simulink model "torch_zdof_sim"  (R2025b)
settings: Solver=VariableStepAuto  StartTime=0.0  StopTime=267.8481  RelTol=1e-3
values from neighbouring files (symbols this model uses):
  framePeriod_s = 1/frameRate_hz    (= 0.005)    [setup.m]
  frameRate_hz = 200    [setup.m]
undefined symbols (not defined in the file or in its folder): Aircraft
libraries: simulink x11, slpidlib x3, uavutilslib x1
settings Model: Creator=amark  LastModifiedBy=zpowe
settings RTWCC: GenCodeOnly=on  Toolchain=MinGW64 | gmake (64-bit Windows)

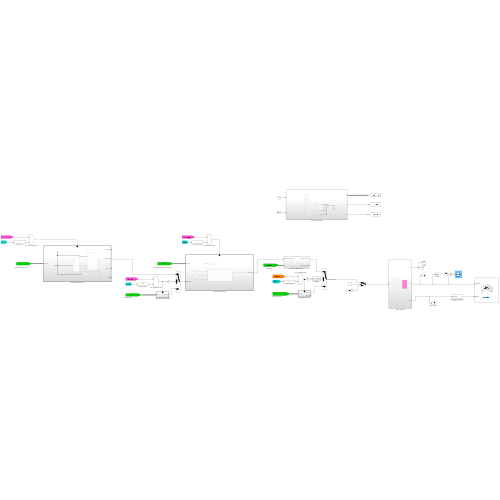
[thumbnail: Simulink's stored preview of the top-level diagram]
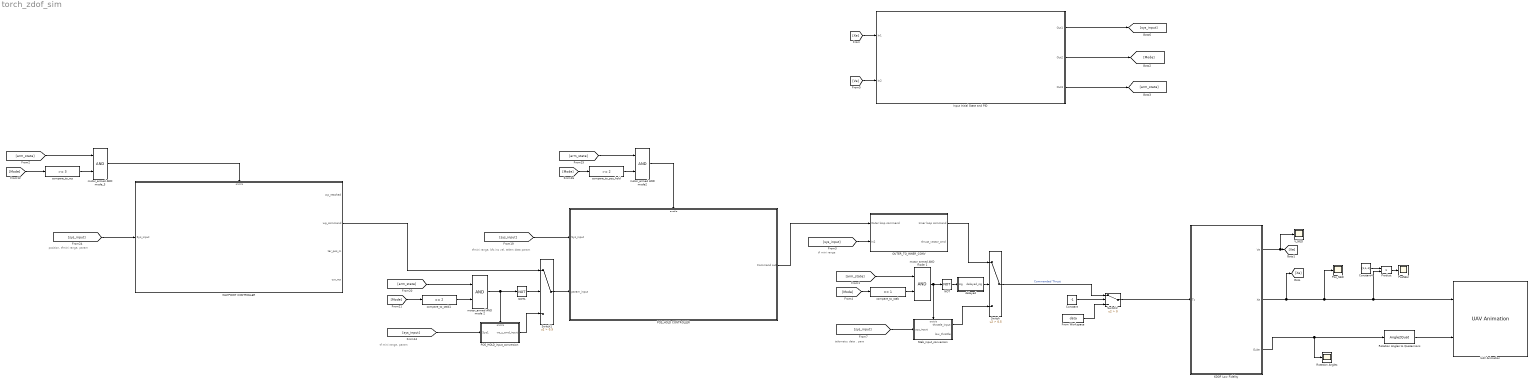
== system torch_zdof_sim ==
  note: position, tfmini range, param
  note: tf mini range, param
  note: tfmini range, bfs ins vel, telem data param
  note: telemetry data . para
  note: tf mini range
  6DOF Low Fidelity : Subsystem
  Constant : Constant  Value=-1
  Constant4 : Constant  Value=[1,1,-1]
  From Workspace : FromWorkspace  VariableName=data  SampleTime=0.005
  Input Initial State and PID : Subsystem
  NOT : Logic  Operator=NOT  IconShape=distinctive  AllPortsSameDT=off  OutDataTypeStr=boolean
  NOT1 : Logic  Operator=NOT  IconShape=distinctive  AllPortsSameDT=off  OutDataTypeStr=boolean
  OUTER_TO_INNER_CONV : Subsystem
  POS_HOLD CONTROLLER : Subsystem
  POS_HOLD_input_conversion : Subsystem
  PosNEU : Scope
      settings: ActiveDisplayYMinimum=-0.21626329278447132  ActiveDisplayYMaximum=2.0187949768508888
  Pos_NED : Scope
      settings: ActiveDisplayYMinimum=-8.6714235476794528  ActiveDisplayYMaximum=15.654477836769015  DataLoggingVariableName=ScopeData7
  Product : Product
  Rotation Angles : Scope
      settings: ActiveDisplayYMinimum=-3.621315177012066  ActiveDisplayYMaximum=3.4944012677530658  DataLoggingVariableName=ScopeData3
  Rotation Angles to Quaternions : Angle2Quat  rotationOrder=XYZ
      settings: AttributesFormatString=Rotation Order: %<rotationOrder>
  Stab_input_conversion : Subsystem
  Switch : Switch  Criteria=u2 > Threshold  Threshold=0.5  SaturateOnIntegerOverflow=off  InputSameDT=off
  Switch1 : Switch  Criteria=u2 > Threshold  Threshold=0.5  SaturateOnIntegerOverflow=off  InputSameDT=off
  Switch2 : Switch  Criteria=u2 > Threshold  SaturateOnIntegerOverflow=off  InputSameDT=off
  UAV Animation : uavutilslib/UAV Animation  NumUAV=1  DynamicUAVConfig=off  UAVType=Multirotor  UAVSize=1  UAVColor=[1 0 0]  UAVTrajectoryAlpha=1  InertialZDirection=Down  RotationFormat=Quaternion  DrawMarkers=off  SampleTime=0.5
  V_NED : Scope
      settings: ActiveDisplayYMinimum=-0.923125150146191  ActiveDisplayYMaximum=0.89093380676990863  DataLoggingVariableName=ScopeData2
  WAYPOINT CONTROLLER : Subsystem
  compare_to_pos_hold : simulink/Logic and Bit Operations/Compare To Constant  relop=>=  const=2  OutDataTypeStr=boolean
  compare_to_stab : simulink/Logic and Bit Operations/Compare To Constant  relop===  const=1  OutDataTypeStr=boolean
  compare_to_stab1 : simulink/Logic and Bit Operations/Compare To Constant  relop===  const=2  OutDataTypeStr=boolean
  compare_to_wp : simulink/Logic and Bit Operations/Compare To Constant  relop=>=  const=3  OutDataTypeStr=boolean
  delayed : Subsystem
  motor_armed AND mode 1 : Logic  IconShape=distinctive  AllPortsSameDT=off  OutDataTypeStr=boolean
  motor_armed AND mode 2 : Logic  IconShape=distinctive  AllPortsSameDT=off  OutDataTypeStr=boolean
  motor_armed AND mode2 : Logic  IconShape=distinctive  AllPortsSameDT=off  OutDataTypeStr=boolean
  motor_armed AND mode_3 : Logic  IconShape=distinctive  AllPortsSameDT=off  OutDataTypeStr=boolean
  wires:
  6DOF Low Fidelity/2(Xe) -> [Xe], UAV Animation/1, Product/2, Pos_NED/1
  6DOF Low Fidelity/1(Ve) -> V_NED/1, [Ve]
  6DOF Low Fidelity/3(Euler) -> Rotation Angles to Quaternions/1, Rotation Angles/1
  Constant4/1 -> Product/1
  Product/1 -> PosNEU/1
  Rotation Angles to Quaternions/1 -> UAV Animation/2
  [sys_input] -> POS_HOLD CONTROLLER/1(Sys_input)
  compare_to_pos_hold/1 -> motor_armed AND mode2/2
  compare_to_wp/1 -> motor_armed AND mode_3/2
  compare_to_stab1/1 -> motor_armed AND mode 2/2
  motor_armed AND mode 2/1 -> NOT1/1, POS_HOLD_input_conversion/Enable
  [arm_state] -> motor_armed AND mode 1/1
  POS_HOLD CONTROLLER/1(Command out) -> OUTER_TO_INNER_CONV/1(Outer loop command)
  compare_to_stab/1 -> motor_armed AND mode 1/2
  [Mode] -> compare_to_wp/1
  [arm_state] -> motor_armed AND mode2/1
  Switch1/1 -> POS_HOLD CONTROLLER/2(param_input)
  Stab_input_conversion/1(throttle_input) -> Switch/3
  [Mode] -> compare_to_stab1/1
  NOT1/1 -> Switch1/2
  [sys_input] -> POS_HOLD_input_conversion/1(Sys1)
  WAYPOINT CONTROLLER/2(wp_command) -> Switch1/1
  [sys_input] -> Stab_input_conversion/1(sys_input)
  delayed/1(delayed_sig) -> Switch/2
  motor_armed AND mode_3/1 -> WAYPOINT CONTROLLER/Enable
  POS_HOLD_input_conversion/1(ve_z_cmd_input) -> Switch1/3
  [arm_state] -> motor_armed AND mode 2/1
  [sys_input] -> OUTER_TO_INNER_CONV/2(In2)
  [sys_input] -> WAYPOINT CONTROLLER/1(Sys_input)
  [Mode] -> compare_to_pos_hold/1
  NOT/1 -> delayed/1(sig)
  [arm_state] -> motor_armed AND mode_3/1
  OUTER_TO_INNER_CONV/1(Inner loop command) -> Switch/1
  motor_armed AND mode 1/1 -> NOT/1, Stab_input_conversion/Enable
  [Mode] -> compare_to_stab/1
  motor_armed AND mode2/1 -> POS_HOLD CONTROLLER/Enable
  Input Initial State and PID/1(Out1) -> [sys_input]
  Input Initial State and PID/2(Out2) -> [Mode]
  Input Initial State and PID/3(Out3) -> [arm_state]
  [Ve] -> Input Initial State and PID/2(In2)
  [Xe] -> Input Initial State and PID/1(In1)
  From Workspace/1 -> Switch2/3
  Switch2/1 -> 6DOF Low Fidelity/1(Tz)
  Constant/1 -> Switch2/2
  Switch/1 -> Switch2/1  "Commanded Thrust"

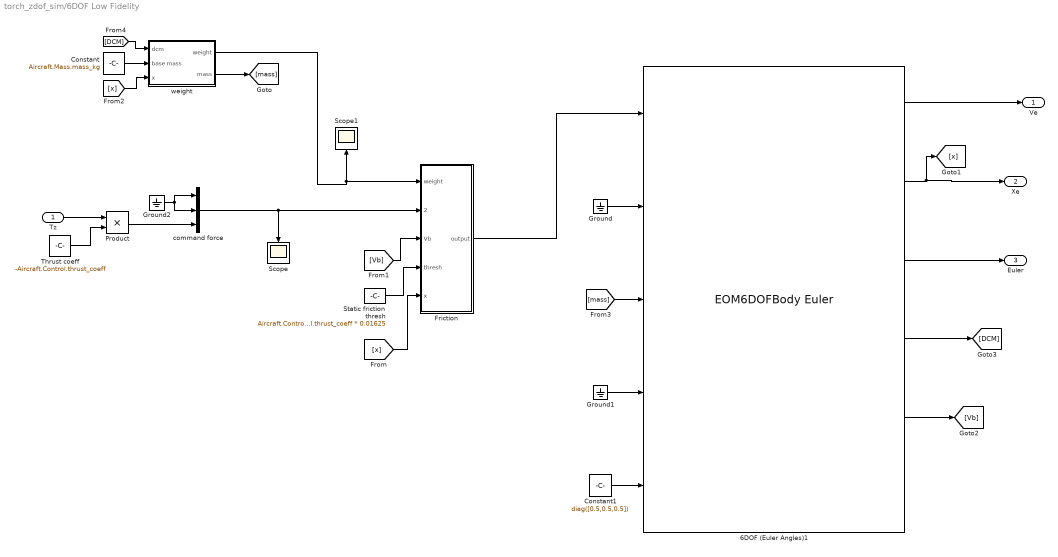
== system torch_zdof_sim/6DOF Low Fidelity ==
  Tz : Inport
  " command force" : Mux  Inputs=3
  6DOF (Euler Angles)1 : EOM6DOFBodyEuler  mtype=Custom Variable  mass_0=Aircraft.Mass.mass_kg  inertia=diag([3.2e-4,100,100])  mass_flag=on
  Constant : Constant  Value=Aircraft.Mass.mass_kg
  Constant1 : Constant  Value=diag([0.5,0.5,0.5])
  Friction : MATLAB Function  TreatAsAtomicUnit=on
  Ground : Ground
  Ground1 : Ground
  Ground2 : Ground
  Product : Product
  Scope : Scope
      settings: ActiveDisplayYMinimum=-1  ActiveDisplayYMaximum=1  DataLoggingVariableName=ScopeData5
  Scope1 : Scope
      settings: ActiveDisplayYMinimum=-12.429607540477818  ActiveDisplayYMaximum=125.41660771198916  DataLoggingVariableName=ScopeData6
  Static friction thresh : Constant  Value=Aircraft.Control.thrust_coeff * 0.01625
  Thrust coeff : Constant  Value=-Aircraft.Control.thrust_coeff
  weight : Subsystem
  Ve : Outport
  Xe : Outport  Port=2
  Euler : Outport  Port=3
  wires:
  6DOF (Euler Angles)1/2 -> [x], Xe/1
  6DOF (Euler Angles)1/3 -> Euler/1
  6DOF (Euler Angles)1/1 -> Ve/1
  6DOF (Euler Angles)1/5 -> [Vb]
  6DOF (Euler Angles)1/4 -> [DCM]
  weight/1(weight) -> Scope1/1, Friction/1(weight)
  " command force"/1 -> Scope/1, Friction/2(F_command)
  [DCM] -> weight/1(dcm)
  [Vb] -> Friction/3(Vb)
  Ground2/1 -> " command force"/2, " command force"/1
  Friction/1(output) -> 6DOF (Euler Angles)1/1
  Tz/1 -> Product/1
  Static friction thresh/1 -> Friction/4(thresh)
  Constant/1 -> weight/2(base mass)
  [x] -> weight/3(x)
  Product/1 -> " command force"/3
  Thrust coeff/1 -> Product/2
  Ground/1 -> 6DOF (Euler Angles)1/2
  [x] -> Friction/5(x)
  Ground1/1 -> 6DOF (Euler Angles)1/4
  weight/2(mass) -> [mass]
  [mass] -> 6DOF (Euler Angles)1/3
  Constant1/1 -> 6DOF (Euler Angles)1/5

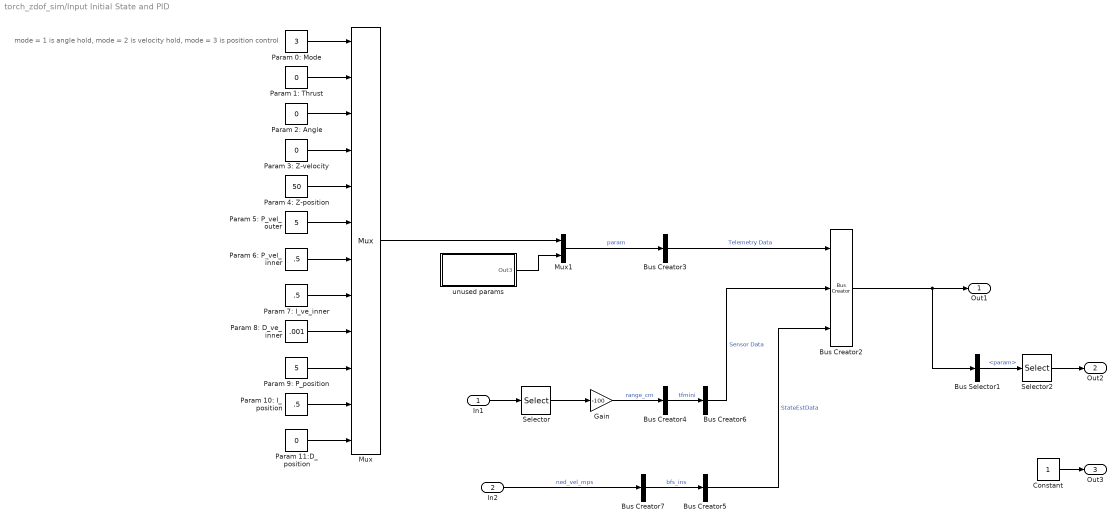
== system torch_zdof_sim/Input Initial State and PID ==
  note: mode = 1 is angle hold, mode = 2 is velocity hold, mode = 3 is position control
  In1 : Inport
  In2 : Inport  Port=2
  Bus Creator2 : BusCreator  Inputs=3
  Bus Creator{3..7} (5 alike) : BusCreator  Inputs=1
  Bus Selector1 : BusSelector  OutputSignals=Telemetry Data.param
  Constant : Constant
  Gain : Gain  Gain=-100
  Mux : Mux  Inputs=12
  Mux1 : Mux  Inputs=2
  Param 0: Mode : Constant  Value=3
  Param 10: I_position : Constant  Value=.5
  Param 11:D_position : Constant  Value=0
  Param 1: Thrust : Constant  Value=0
  Param 2: Angle : Constant  Value=0
  Param 3: Z-velocity : Constant  Value=0
  Param 4: Z-position : Constant  Value=50
  Param 5: P_vel_outer : Constant  Value=5
  Param 6: P_vel_inner : Constant  Value=.5
  Param 7: I_ve_inner : Constant  Value=.5
  Param 8: D_ve_inner : Constant  Value=.001
  Param 9: P_position : Constant  Value=5
  Selector : Selector  InputPortWidth=3  IndexOptions=Index vector (dialog)  Indices=[3]  OutputSizes=1
  Selector2 : Selector  IndexMode=Zero-based  InputPortWidth=24  IndexOptions=Index vector (dialog)  Indices=0  OutputSizes=1
  unused params : Subsystem
  Out1 : Outport
  Out2 : Outport  Port=2
  Out3 : Outport  Port=3
  wires:
  Param 3: Z-velocity/1 -> Mux/4
  Bus Creator5/1 -> Bus Creator2/3  "StateEstData"
  Param 2: Angle/1 -> Mux/3
  Param 4: Z-position/1 -> Mux/5
  Selector/1 -> Gain/1
  Param 11:D_position/1 -> Mux/12
  Param 10: I_position/1 -> Mux/11
  Param 9: P_position/1 -> Mux/10
  Bus Creator6/1 -> Bus Creator2/2  "Sensor Data"
  Param 7: I_ve_inner/1 -> Mux/8
  Param 1: Thrust/1 -> Mux/2
  Param 5: P_vel_outer/1 -> Mux/6
  Bus Creator4/1 -> Bus Creator6/1  "tfmini"
  Bus Creator3/1 -> Bus Creator2/1  "Telemetry Data"
  Param 8: D_ve_inner/1 -> Mux/9
  Param 0: Mode/1 -> Mux/1
  Gain/1 -> Bus Creator4/1  "range_cm"
  Param 6: P_vel_inner/1 -> Mux/7
  In1/1 -> Selector/1
  In2/1 -> Bus Creator7/1  "ned_vel_mps"
  Mux/1 -> Mux1/1
  Bus Creator7/1 -> Bus Creator5/1  "bfs_ins"
  Bus Selector1/1 -> Selector2/1  "<param>"
  Bus Creator2/1 -> Bus Selector1/1, Out1/1
  Selector2/1 -> Out2/1
  Constant/1 -> Out3/1
  Mux1/1 -> Bus Creator3/1  "param"
  unused params/1(Out3) -> Mux1/2

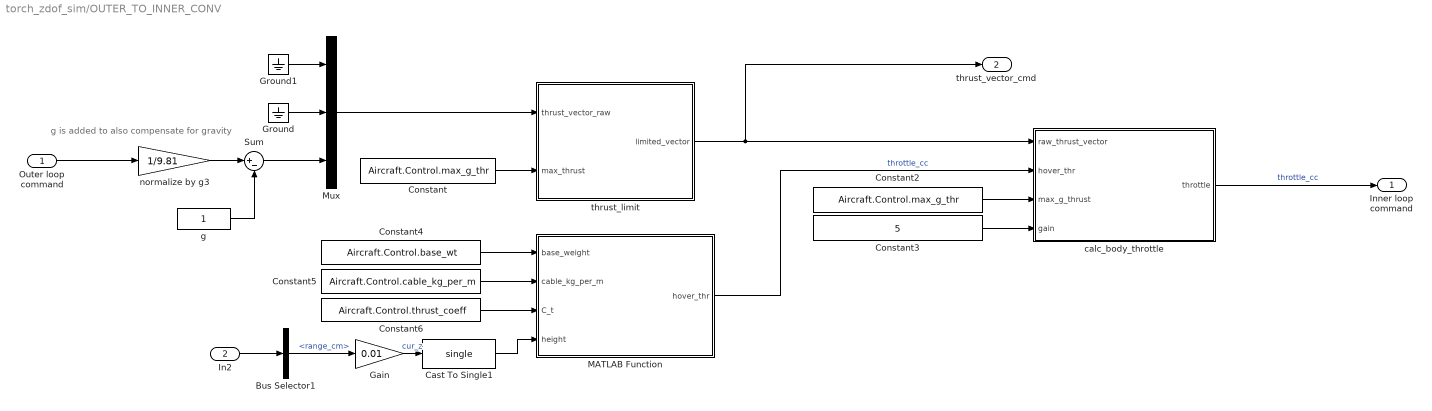
== system torch_zdof_sim/OUTER_TO_INNER_CONV ==
  note: g is added to also compensate for gravity
  Outer loop command : Inport
  In2 : Inport  Port=2
  Bus Selector1 : BusSelector  OutputSignals=Sensor Data.tfmini.range_cm
  Cast To Single1 : DataTypeConversion  OutDataTypeStr=single  SaturateOnIntegerOverflow=off  RndMeth=Floor
  Constant : Constant  Value=Aircraft.Control.max_g_thr  OutDataTypeStr=single
  Constant2 : Constant  Value=Aircraft.Control.max_g_thr  OutDataTypeStr=single
  Constant3 : Constant  Value=5  OutDataTypeStr=single
  Constant4 : Constant  Value=Aircraft.Control.base_wt  OutDataTypeStr=double
  Constant5 : Constant  Value=Aircraft.Control.cable_kg_per_m  OutDataTypeStr=double
  Constant6 : Constant  Value=Aircraft.Control.thrust_coeff  OutDataTypeStr=double
  Gain : Gain  Gain=0.01
  Ground : Ground
  Ground1 : Ground
  MATLAB Function : MATLAB Function  TreatAsAtomicUnit=on
  Mux : Mux  Inputs=3
  Sum : Sum  Inputs=|+-
  calc_body_throttle : MATLAB Function  TreatAsAtomicUnit=on
  g : Constant  OutDataTypeStr=single
  normalize by g3 : Gain  Gain=1/9.81
  thrust_limit : MATLAB Function  TreatAsAtomicUnit=on
  Inner loop command : Outport
  thrust_vector_cmd : Outport  Port=2
  wires:
  Constant/1 -> thrust_limit/2(max_thrust)
  Mux/1 -> thrust_limit/1(thrust_vector_raw)
  Outer loop command/1 -> normalize by g3/1
  g/1 -> Sum/2
  normalize by g3/1 -> Sum/1
  Ground1/1 -> Mux/1
  Ground/1 -> Mux/2
  Sum/1 -> Mux/3
  calc_body_throttle/1(throttle) -> Inner loop command/1  "throttle_cc"
  thrust_limit/1(limited_vector) -> calc_body_throttle/1(raw_thrust_vector), thrust_vector_cmd/1
  Constant2/1 -> calc_body_throttle/3(max_g_thrust)
  Constant3/1 -> calc_body_throttle/4(gain)
  Constant5/1 -> MATLAB Function/2(cable_kg_per_m)
  In2/1 -> Bus Selector1/1
  Bus Selector1/1 -> Gain/1  "<range_cm>"
  Constant6/1 -> MATLAB Function/3(C_t)
  MATLAB Function/1(hover_thr) -> calc_body_throttle/2(hover_thr)  "throttle_cc"
  Cast To Single1/1 -> MATLAB Function/4(height)
  Gain/1 -> Cast To Single1/1  "cur_z"
  Constant4/1 -> MATLAB Function/1(base_weight)

== system torch_zdof_sim/POS_HOLD CONTROLLER ==
  Sys_input : Inport
  param_input : Inport  Port=2
  Enable : EnablePort  StatesWhenEnabling=reset  PropagateVarSize=During execution  ShowOutputPort=on
  Vertical speed controller : Subsystem
  Command out : Outport
  wires:
  Enable/1 -> [pos_hold_init]
  Vertical speed controller/1(acc_z_cmd) -> Command out/1  "acc_z_cmd"
  Sys_input/1 -> Vertical speed controller/3(sys_data)
  [pos_hold_init] -> Vertical speed controller/2(pos_hold_init)
  param_input/1 -> Vertical speed controller/1(ve_z_cmd_mps)

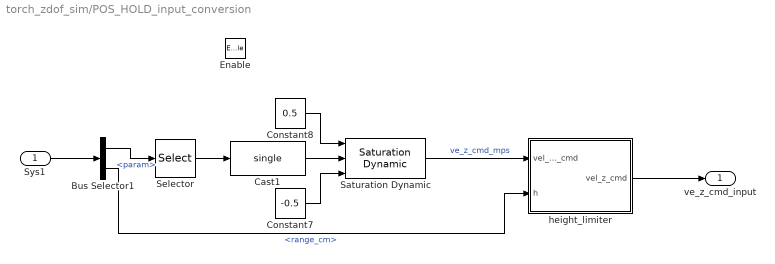
== system torch_zdof_sim/POS_HOLD_input_conversion ==
  Sys1 : Inport
  Enable : EnablePort
  Bus Selector1 : BusSelector  OutputSignals=Telemetry Data.param,Sensor Data.tfmini.range_cm
  Cast1 : DataTypeConversion  OutDataTypeStr=single  SaturateOnIntegerOverflow=off  RndMeth=Floor
  Constant7 : Constant  Value=-0.5
  Constant8 : Constant  Value=0.5
  Saturation Dynamic : simulink/Discontinuities/Saturation Dynamic  OutMin=[]  OutMax=[]  OutDataTypeStr=double  OutDataType=fixdt(1, 16)  OutScaling=2^-10  DoSatur=off
  Selector : Selector  IndexMode=Zero-based  InputPortWidth=24  IndexOptions=Index vector (dialog)  Indices=3  OutputSizes=1
  height_limiter : MATLAB Function  TreatAsAtomicUnit=on
  ve_z_cmd_input : Outport
  wires:
  Sys1/1 -> Bus Selector1/1
  Constant8/1 -> Saturation Dynamic/1
  Constant7/1 -> Saturation Dynamic/3
  Bus Selector1/1 -> Selector/1  "<param>"
  Cast1/1 -> Saturation Dynamic/2
  Selector/1 -> Cast1/1
  Saturation Dynamic/1 -> height_limiter/1(vel_param_cmd)  "ve_z_cmd_mps"
  Bus Selector1/2 -> height_limiter/2(h)  "<range_cm>"
  height_limiter/1(vel_z_cmd) -> ve_z_cmd_input/1

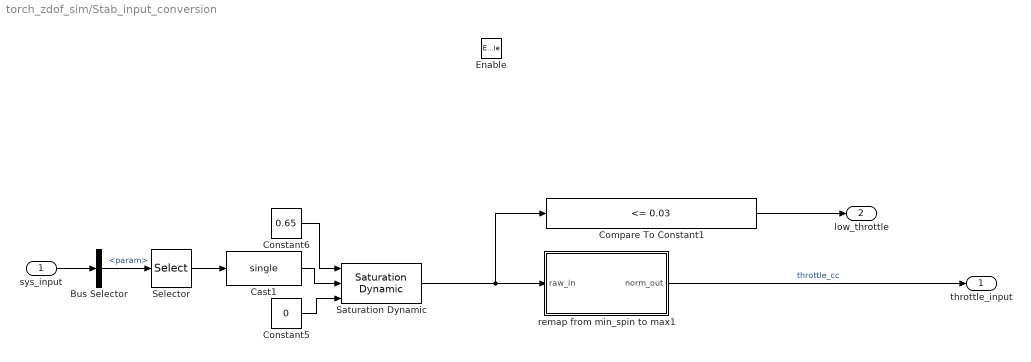
== system torch_zdof_sim/Stab_input_conversion ==
  sys_input : Inport
  Enable : EnablePort
  Bus Selector : BusSelector  OutputSignals=Telemetry Data.param
  Cast1 : DataTypeConversion  OutDataTypeStr=single  SaturateOnIntegerOverflow=off  RndMeth=Floor
  Compare To Constant1 : simulink/Logic and Bit Operations/Compare To Constant  relop=<=  const=0.03  OutDataTypeStr=boolean
  Constant5 : Constant  Value=0
  Constant6 : Constant  Value=0.65
  Saturation Dynamic : simulink/Discontinuities/Saturation Dynamic  OutMin=[]  OutMax=[]  OutDataTypeStr=double  OutDataType=fixdt(1, 16)  OutScaling=2^-10  DoSatur=off
  Selector : Selector  IndexMode=Zero-based  InputPortWidth=24  IndexOptions=Index vector (dialog)  Indices=1  OutputSizes=1
  remap from min_spin to max1 : Subsystem
  throttle_input : Outport
  low_throttle : Outport  Port=2
  wires:
  Compare To Constant1/1 -> low_throttle/1
  Constant6/1 -> Saturation Dynamic/1
  sys_input/1 -> Bus Selector/1
  Cast1/1 -> Saturation Dynamic/2
  Selector/1 -> Cast1/1
  Constant5/1 -> Saturation Dynamic/3
  Bus Selector/1 -> Selector/1  "<param>"
  Saturation Dynamic/1 -> Compare To Constant1/1, remap from min_spin to max1/1(raw_in)
  remap from min_spin to max1/1(norm_out) -> throttle_input/1  "throttle_cc"

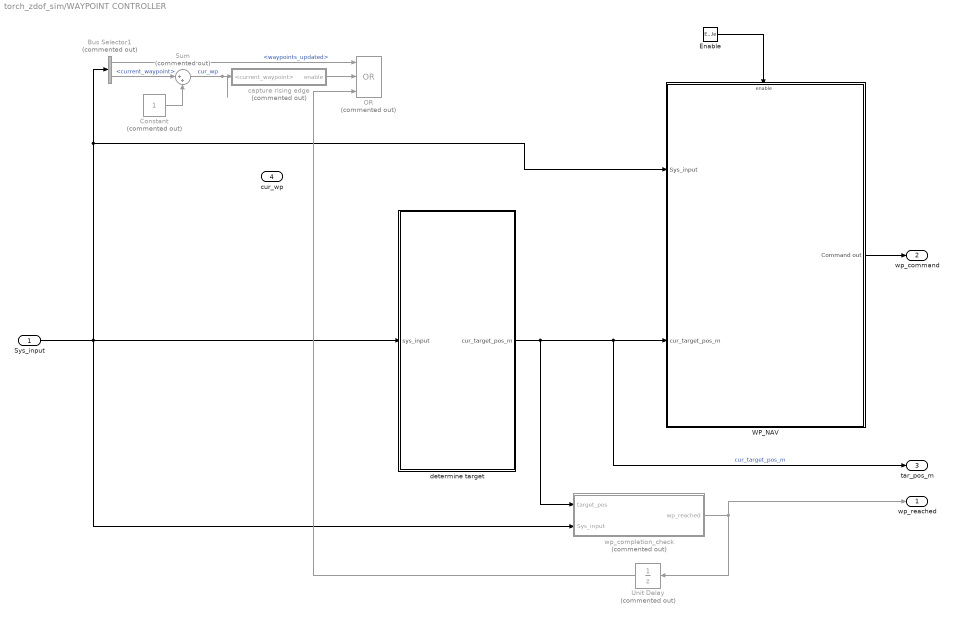
== system torch_zdof_sim/WAYPOINT CONTROLLER ==
  Sys_input : Inport
  Enable : EnablePort  StatesWhenEnabling=reset  ShowOutputPort=on
  Bus Selector1 : BusSelector  Commented=on  OutputSignals=Telemetry Data.waypoints_updated,Telemetry Data.current_waypoint
  Constant : Constant  Commented=on  OutDataTypeStr=int16
  OR : Logic  Commented=on  Operator=OR  Inputs=3  IconShape=distinctive  AllPortsSameDT=off  OutDataTypeStr=boolean
  Sum : Sum  Commented=on  Inputs=|++
  Unit Delay : UnitDelay  Commented=on  SampleTime=-1  HasFrameUpgradeWarning=on
  WP_NAV : Subsystem
  capture rising edge : Subsystem  Commented=on
  determine target : Subsystem
  wp_completion_check : Subsystem  Commented=on
  wp_reached : Outport
  wp_command : Outport  Port=2
  tar_pos_m : Outport  Port=3
  cur_wp : Outport  Port=4
  wires:
  Sys_input/1 -> Bus Selector1/1, WP_NAV/1(Sys_input), wp_completion_check/2(Sys_input), determine target/1(sys_input)
  Enable/1 -> WP_NAV/Enable
  WP_NAV/1(Command out) -> wp_command/1
  determine target/1(cur_target_pos_m) -> tar_pos_m/1, WP_NAV/2(cur_target_pos_m), wp_completion_check/1(target_pos)  "cur_target_pos_m"
  Bus Selector1/1 -> OR/1  "<waypoints_updated>"
  capture rising edge/1(enable) -> OR/2
  Unit Delay/1 -> OR/3
  wp_completion_check/1(wp_reached) -> wp_reached/1, Unit Delay/1
  Constant/1 -> Sum/2
  Bus Selector1/2 -> Sum/1  "<current_waypoint>"
  Sum/1 -> capture rising edge/1(<current_waypoint>)  "cur_wp"

== system torch_zdof_sim/delayed ==
  sig : Inport
  Constant : Constant  Value=framePeriod_s  OutDataTypeStr=double
  Constant1 : Constant  Value=0.5  OutDataTypeStr=single
  Delay : Delay  DelayLengthSource=Input port
      settings: InputPortMap=u0,p1
  Divide : Product  Inputs=*/
  delayed_sig : Outport
  wires:
  Delay/1 -> delayed_sig/1
  sig/1 -> Delay/1
  Divide/1 -> Delay/2
  Constant/1 -> Divide/2
  Constant1/1 -> Divide/1

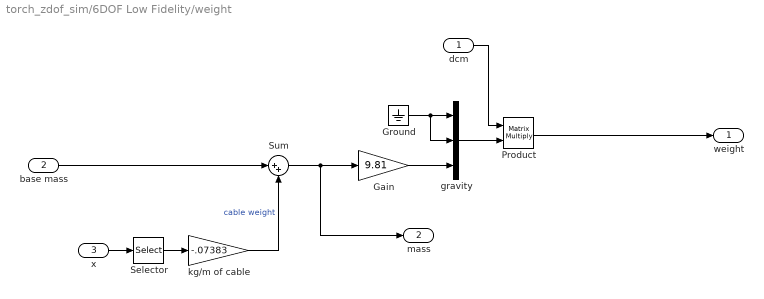
== system torch_zdof_sim/6DOF Low Fidelity/weight ==
  dcm : Inport
  base mass : Inport  Port=2
  x : Inport  Port=3
  Gain : Gain  Gain=9.81
  Ground : Ground
  Product : Product  Multiplication=Matrix(*)
  Selector : Selector  InputPortWidth=3  IndexOptions=Index vector (dialog)  Indices=[3]  OutputSizes=1
  Sum : Sum  Inputs=|++
  gravity : Mux  Inputs=3
  kg/m of cable : Gain  Gain=-.07383
  weight : Outport
  mass : Outport  Port=2
  wires:
  Ground/1 -> gravity/2, gravity/1
  gravity/1 -> Product/2
  base mass/1 -> Sum/1
  dcm/1 -> Product/1
  Gain/1 -> gravity/3
  Product/1 -> weight/1
  Sum/1 -> mass/1, Gain/1
  x/1 -> Selector/1
  Selector/1 -> kg/m of cable/1
  kg/m of cable/1 -> Sum/2  "cable weight"

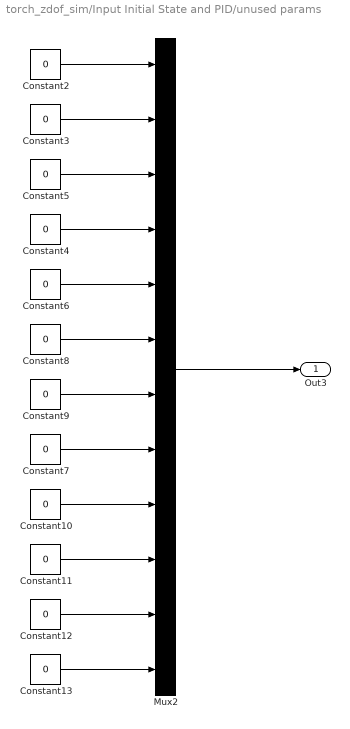
== system torch_zdof_sim/Input Initial State and PID/unused params ==
  Constant{2..13} (12 alike) : Constant  Value=0
  Mux2 : Mux  Inputs=12
  Out3 : Outport
  wires:
  Mux2/1 -> Out3/1
  Constant13/1 -> Mux2/12
  Constant12/1 -> Mux2/11
  Constant11/1 -> Mux2/10
  Constant10/1 -> Mux2/9
  Constant9/1 -> Mux2/7
  Constant8/1 -> Mux2/6
  Constant7/1 -> Mux2/8
  Constant6/1 -> Mux2/5
  Constant5/1 -> Mux2/3
  Constant4/1 -> Mux2/4
  Constant3/1 -> Mux2/2
  Constant2/1 -> Mux2/1

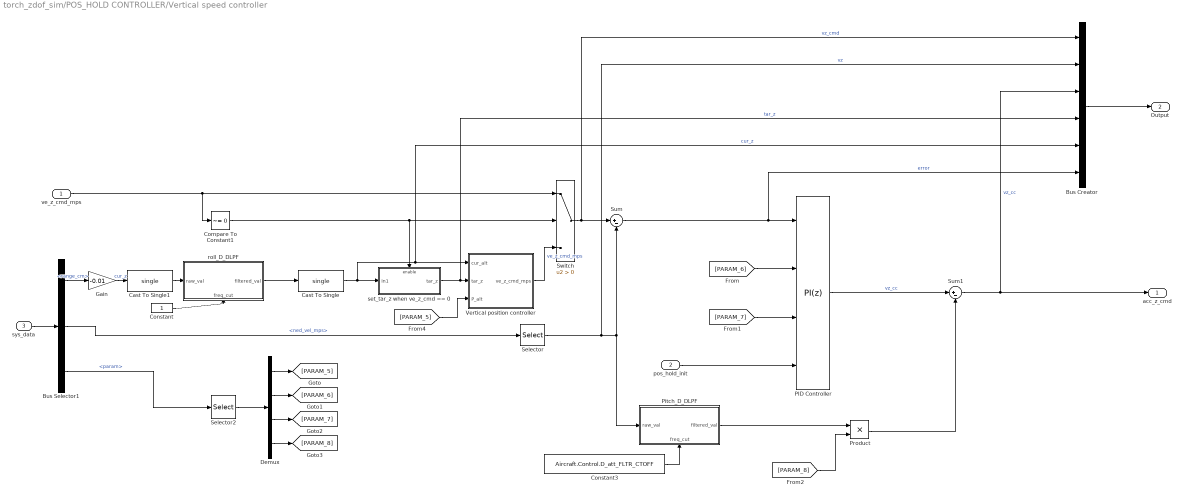
== system torch_zdof_sim/POS_HOLD CONTROLLER/Vertical speed controller ==
  ve_z_cmd_mps : Inport
  pos_hold_init : Inport  Port=2
  sys_data : Inport  Port=3
  Bus Creator : BusCreator  Inputs=6
  Bus Selector1 : BusSelector  OutputSignals=Sensor Data.tfmini.range_cm,StateEstData.bfs_ins.ned_vel_mps,Telemetry Data.param
  Cast To Single : DataTypeConversion  OutDataTypeStr=single  SaturateOnIntegerOverflow=off  RndMeth=Floor
  Cast To Single1 : DataTypeConversion  OutDataTypeStr=single  SaturateOnIntegerOverflow=off  RndMeth=Floor
  Compare To Constant1 : simulink/Logic and Bit Operations/Compare To Constant  relop=~=  const=0  OutDataTypeStr=boolean
  Constant : Constant  OutDataTypeStr=single
  Constant3 : Constant  Value=Aircraft.Control.D_att_FLTR_CTOFF  OutDataTypeStr=single
  Demux : Demux
  Gain : Gain  Gain=-0.01
  PID Controller : slpidlib/PID Controller  Controller=PI  Form=Parallel  TimeDomain=Discrete-time  UseExternalTs=off  SampleTime=framePeriod_s  IntegratorMethod=Forward Euler  FilterMethod=Forward Euler  ControllerParametersSource=external  P=0  I=0  UseKiTs=off  D=0  UseExternalDerivativeSource=off  N=100  UseFilter=off  TunerSelectOption=Frequency Response Based  InitialConditionSource=internal  InitialConditionForIntegrator=0  InitialConditionForFilter=0  DifferentiatorICPrevScaledInput=0  ExternalReset=either  TrackingMode=off  Kt=1  LimitOutput=on  SatLimitsSource=internal  UpperSaturationLimit=1  LowerSaturationLimit=-1  LinearizeAsGain=on  AntiWindupMode=clamping  Kb=1  LimitIntegrator=off  UpperIntegratorSaturationLimit=inf  LowerIntegratorSaturationLimit=-inf  POutMin=[]  POutMax=[]  IOutMin=[]  IOutMax=[]  DOutMin=[]  DOutMax=[]  NOutMin=[]  NOutMax=[]  SumOutMin=[]  SumOutMax=[]  SaturationOutMin=[]  SaturationOutMax=[]  PParamMin=[]  PParamMax=[]  IParamMin=[]  IParamMax=[]  DParamMin=[]  DParamMax=[]  NParamMin=[]  NParamMax=[]  KbParamMin=[]  KbParamMax=[]  KtParamMin=[]  KtParamMax=[]  KbOutMin=[]  KbOutMax=[]  KtOutMin=[]  KtOutMax=[]  IntegratorOutMin=[]  IntegratorOutMax=[]  FilterOutMin=[]  FilterOutMax=[]  SumI1OutMin=[]  SumI1OutMax=[]  SumI2OutMin=[]  SumI2OutMax=[]  SumI3OutMin=[]  SumI3OutMax=[]  SumI4OutMin=[]  SumI4OutMax=[]  SumDOutMin=[]  SumDOutMax=[]  DifferentiatorOutMin=[]  DifferentiatorOutMax=[]  FilterDiffOutCoefMin=[]  FilterDiffOutCoefMax=[]  ReciprocalOutMin=[]  ReciprocalOutMax=[]  SumDenOutMin=[]  SumDenOutMax=[]  SumNumOutMin=[]  SumNumOutMax=[]  DivideOutMin=[]  DivideOutMax=[]  UdiffTsProdOutMin=[]  UdiffTsProdOutMax=[]  NTsProdOutMin=[]  NTsProdOutMax=[]  UintegralTsProdOutMin=[]  UintegralTsProdOutMax=[]  UngainTsProdOutMin=[]  UngainTsProdOutMax=[]  ClampingZeroOutDataTypeStr=Inherit: Inherit via back propagation  ClampingZeroOutMin=[]  ClampingZeroOutMax=[]  FilterDenConstantOutDataTypeStr=Inherit: Inherit via back propagation  FilterDenConstantOutMin=[]  FilterDenConstantOutMax=[]  PCopyOutDataTypeStr=Inherit: Inherit via back propagation  PCopyOutMin=[]  PCopyOutMax=[]  NCopyOutDataTypeStr=Inherit: Inherit via back propagation  NCopyOutMin=[]  NCopyOutMax=[]  IntegratorContinuousStateAttributes=''  IntegratorStateMustResolveToSignalObject=off  IntegratorRTWStateStorageClass=Auto  FilterContinuousStateAttributes=''  FilterStateMustResolveToSignalObject=off  FilterRTWStateStorageClass=Auto  ParallelPVariant=ExternalParameters  IdealPVariant=Disabled  IVariant=ExternalParameters  DVariant=Disabled  IntegratorVariant=Discrete  SatVariant=Enabled  AWVariant=DiscClampingParallel  PCopyVariant=Disabled  TRVariant=Disabled  FdbkBlocksVariant=Forward  IdealPFdbkVariant=Disabled  SatFdbkVariant=Disabled  DerivativeFilterVariant=Disabled  NVariant=Disabled  NCopyVariant=Disabled_SignalSpec  FilterICVariant=Disabled  IntegratorICVariant=InternalICs  ExternalResetVariant=ExternalReset  TRSumVariant=Passthrough  SumFdbkVariant=Disabled  SumVariant=Sum_PI  TsampFilterVariant=InternalTs  TsampNgainVariant=Passthrough  TsampIntegralVariant=Disabled_SignalSpec  ExternalSaturationOutDataTypeStr=Inherit: Same as second input  DerivativeSourceVariant=Disabled  PreIntVariant=InternalPreInt
  Pitch_D_DLPF : Subsystem
      settings: PortSchema="{\"entries\":[{\"content\":{\"sides\":[{\"content\":{\"connectorIds\":[\"In1\"]},\"type\":\"ConnectorPlacement.EquallySpacedRectSide\",\"uuid\":\"20236834-aeb3-4c5b-bb2e-f84447e752b5\"},{\"content\":{\"connectorIds\":[\"Out1\"],\"side\":\"RIGHT\"},\"type\":\"ConnectorPlacement.EquallySpacedRectSide\",\"uuid\":\"d668f9a1-a3df-4207-8bf1-99fb838e59b2\"},{\"content\":{\"connectorIds\":[],\"side\":\"TOP\"},\"type\":\"ConnectorPlacement.EquallySpacedRectSide\",\"uuid\":\"66cceb06-f4bc-4278-b965-2427292e46df\"},{\"content\":{\"connectorIds\":[\"In2\"],\"side\":\"BOTTOM\"},\"type\":\"ConnectorPlacement.EquallySpacedRectSide\",\"uuid\":\"7d08bc25-8e2d-44c6-8f94-b04e75c70268\"}]},\"type\":\"ConnectorPlacement.EquallySpacedConnector\",\"uuid\":\"3dc29a9a-e794-478d-b7df-452e6c2d3f66\"}],\"packageUris\":[\"http://schema.mathworks.com/mf0/Connector/R2020b\"],\"version\":\"1.0\"}"
  Product : Product
  Selector : Selector  InputPortWidth=3  IndexOptions=Index vector (dialog)  Indices=[3]  OutputSizes=1
  Selector2 : Selector  IndexMode=Zero-based  InputPortWidth=24  IndexOptions=Index vector (dialog)  Indices=[5 6 7 8]  OutputSizes=1
  Sum : Sum  Inputs=|+-
  Sum1 : Sum  Inputs=|+-
  Switch : Switch  Criteria=u2 > Threshold  SaturateOnIntegerOverflow=off  InputSameDT=off
  Vertical position controller : Subsystem
  roll_D_DLPF : Subsystem
      settings: PortSchema="{\"entries\":[{\"content\":{\"sides\":[{\"content\":{\"connectorIds\":[\"In1\"]},\"type\":\"ConnectorPlacement.EquallySpacedRectSide\",\"uuid\":\"20236834-aeb3-4c5b-bb2e-f84447e752b5\"},{\"content\":{\"connectorIds\":[\"Out1\"],\"side\":\"RIGHT\"},\"type\":\"ConnectorPlacement.EquallySpacedRectSide\",\"uuid\":\"d668f9a1-a3df-4207-8bf1-99fb838e59b2\"},{\"content\":{\"connectorIds\":[],\"side\":\"TOP\"},\"type\":\"ConnectorPlacement.EquallySpacedRectSide\",\"uuid\":\"66cceb06-f4bc-4278-b965-2427292e46df\"},{\"content\":{\"connectorIds\":[\"In2\"],\"side\":\"BOTTOM\"},\"type\":\"ConnectorPlacement.EquallySpacedRectSide\",\"uuid\":\"8fdaac6a-cb03-4bd4-87bb-7bafd10bc297\"}]},\"type\":\"ConnectorPlacement.EquallySpacedConnector\",\"uuid\":\"3dc29a9a-e794-478d-b7df-452e6c2d3f66\"}],\"packageUris\":[\"http://schema.mathworks.com/mf0/Connector/R2020b\"],\"version\":\"1.0\"}"
  set_tar_z when ve_z_cmd == 0 : Subsystem  TreatAsAtomicUnit=on
  acc_z_cmd : Outport
  Output : Outport  Port=2
  wires:
  [PARAM_6] -> PID Controller/2
  Bus Selector1/2 -> Selector/1  "<ned_vel_mps>"
  sys_data/1 -> Bus Selector1/1
  Pitch_D_DLPF/1(filtered_val) -> Product/1
  Selector/1 -> Bus Creator/2, Sum/2, Pitch_D_DLPF/1(raw_val)  "vz"
  [PARAM_8] -> Product/2
  Product/1 -> Sum1/2
  ve_z_cmd_mps/1 -> Compare To Constant1/1, Switch/1
  Switch/1 -> Bus Creator/1, Sum/1  "vz_cmd"
  set_tar_z when ve_z_cmd == 0/1(tar_z) -> Bus Creator/4, Vertical position controller/2(tar_z)  "tar_z"
  pos_hold_init/1 -> PID Controller/4
  Constant3/1 -> Pitch_D_DLPF/2(freq_cut)
  [PARAM_5] -> Vertical position controller/3(P_alt)
  Bus Creator/1 -> Output/1
  Cast To Single/1 -> Bus Creator/5, Vertical position controller/1(cur_alt), set_tar_z when ve_z_cmd == 0/1(In1)  "cur_z"
  Sum/1 -> Bus Creator/6, PID Controller/1  "error"
  Sum1/1 -> acc_z_cmd/1, Bus Creator/3  "vz_cc"
  PID Controller/1 -> Sum1/1  "vz_cc"
  Bus Selector1/3 -> Selector2/1  "<param>"
  Selector2/1 -> Demux/1
  Demux/1 -> [PARAM_5]
  Demux/2 -> [PARAM_6]
  Demux/3 -> [PARAM_7]
  Demux/4 -> [PARAM_8]
  [PARAM_7] -> PID Controller/3
  Vertical position controller/1(ve_z_cmd_mps) -> Switch/3  "ve_z_cmd_mps"
  Compare To Constant1/1 -> Switch/2, set_tar_z when ve_z_cmd == 0/Enable
  roll_D_DLPF/1(filtered_val) -> Cast To Single/1
  Constant/1 -> roll_D_DLPF/2(freq_cut)
  Bus Selector1/1 -> Gain/1  "<range_cm>"
  Cast To Single1/1 -> roll_D_DLPF/1(raw_val)
  Gain/1 -> Cast To Single1/1  "cur_z"

== system torch_zdof_sim/Stab_input_conversion/remap from min_spin to max1 ==
  raw_in : Inport
  Constant4 : Constant  Value=0  OutDataTypeStr=single
  Constant5 : Constant  Value=Aircraft.Control.motor_spin_min  OutDataTypeStr=double
  Constant6 : Constant  Value=0.8  OutDataTypeStr=double
  Constant7 : Constant  OutDataTypeStr=single
  remap1 : MATLAB Function  TreatAsAtomicUnit=on
  norm_out : Outport
  wires:
  Constant6/1 -> remap1/5(out_max)
  Constant5/1 -> remap1/4(out_min)
  remap1/1(norm_out) -> norm_out/1
  Constant4/1 -> remap1/2(in_min)
  Constant7/1 -> remap1/3(in_max)
  raw_in/1 -> remap1/1(raw_in)

== system torch_zdof_sim/WAYPOINT CONTROLLER/WP_NAV ==
  Sys_input : Inport
  cur_target_pos_m : Inport  Port=2
  Enable : EnablePort  StatesWhenEnabling=reset  PropagateVarSize=During execution  ShowOutputPort=on
  Selector : Selector  InputPortWidth=3  IndexOptions=Index vector (dialog)  Indices=3  OutputSizes=1
  Vertical position controller1 : Subsystem
  Command out : Outport
  wires:
  Vertical position controller1/1(ve_z_cmd_mps) -> Command out/1  "ve_z_cmd_mps"
  cur_target_pos_m/1 -> Selector/1
  Selector/1 -> Vertical position controller1/2(tar_z)
  Sys_input/1 -> Vertical position controller1/1(cur_alt)
  Enable/1 -> Vertical position controller1/3(waypoint_init)

== system torch_zdof_sim/WAYPOINT CONTROLLER/capture rising edge ==
  <current_waypoint> : Inport
  Detect Change1 : simulink/Logic and Bit Operations/Detect Change  vinit=-1  OutDataTypeStr=boolean
  Detect Rise Positive : simulink/Logic and Bit Operations/Detect Rise Positive  Commented=through  vinit=0  OutDataTypeStr=boolean
  enable : Outport
  wires:
  <current_waypoint>/1 -> Detect Change1/1
  Detect Rise Positive/1 -> enable/1
  Detect Change1/1 -> Detect Rise Positive/1

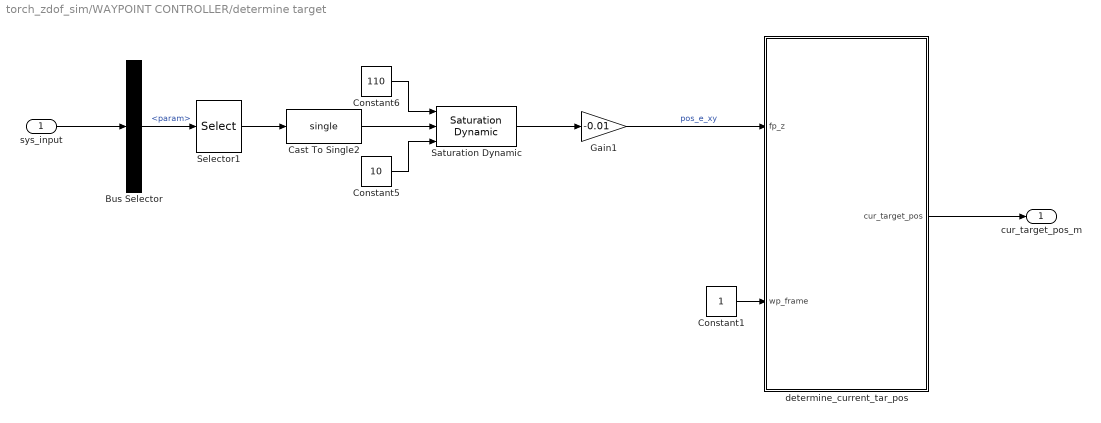
== system torch_zdof_sim/WAYPOINT CONTROLLER/determine target ==
  sys_input : Inport
  Bus Selector : BusSelector  OutputSignals=Telemetry Data.param
  Cast To Single2 : DataTypeConversion  OutDataTypeStr=single  SaturateOnIntegerOverflow=off  RndMeth=Floor
  Constant1 : Constant  OutDataTypeStr=uint8
  Constant5 : Constant  Value=10
  Constant6 : Constant  Value=110
  Gain1 : Gain  Gain=-0.01
  Saturation Dynamic : simulink/Discontinuities/Saturation Dynamic  OutMin=[]  OutMax=[]  OutDataTypeStr=double  OutDataType=fixdt(1, 16)  OutScaling=2^-10  DoSatur=off
  Selector1 : Selector  IndexMode=Zero-based  InputPortWidth=24  IndexOptions=Index vector (dialog)  Indices=4  OutputSizes=1
  determine_current_tar_pos : MATLAB Function  TreatAsAtomicUnit=on
  cur_target_pos_m : Outport
  wires:
  sys_input/1 -> Bus Selector/1
  Constant1/1 -> determine_current_tar_pos/2(wp_frame)
  determine_current_tar_pos/1(cur_target_pos) -> cur_target_pos_m/1
  Bus Selector/1 -> Selector1/1  "<param>"
  Cast To Single2/1 -> Saturation Dynamic/2
  Constant5/1 -> Saturation Dynamic/3
  Constant6/1 -> Saturation Dynamic/1
  Selector1/1 -> Cast To Single2/1
  Saturation Dynamic/1 -> Gain1/1
  Gain1/1 -> determine_current_tar_pos/1(fp_z)  "pos_e_xy"

== system torch_zdof_sim/WAYPOINT CONTROLLER/wp_completion_check ==
  note: Output wp_reached cmd only when distance between current pos and target pos is less than wp_radius.
  target_pos : Inport
  Sys_input : Inport  Port=2
  Bus Selector : BusSelector  OutputSignals=StateEstData.aux_ins.ned_pos_m
  Constant : Constant  Value=Aircraft.Control.wp_radius  OutDataTypeStr=single
  check_wp_reached : MATLAB Function  TreatAsAtomicUnit=on
  wp_reached : Outport
  wires:
  Sys_input/1 -> Bus Selector/1
  Bus Selector/1 -> check_wp_reached/2(ned_pos)  "<ned_pos_m>"
  check_wp_reached/1(reached) -> wp_reached/1
  target_pos/1 -> check_wp_reached/1(target_pos)
  Constant/1 -> check_wp_reached/3(Aircraft_Control_wp_radius)

== system torch_zdof_sim/POS_HOLD CONTROLLER/Vertical speed controller/Pitch_D_DLPF ==
  raw_val : Inport
  freq_cut : Inport  Port=2
  Cast To Double : DataTypeConversion  OutDataTypeStr=double  SaturateOnIntegerOverflow=off  RndMeth=Floor
  Cast To Double1 : DataTypeConversion  OutDataTypeStr=double  SaturateOnIntegerOverflow=off  RndMeth=Floor
  MATLAB Function : MATLAB Function  TreatAsAtomicUnit=on
  Unit Delay : UnitDelay  SampleTime=-1  HasFrameUpgradeWarning=on
  filtered_val : Outport
  wires:
  MATLAB Function/1(filtered_val) -> filtered_val/1, Unit Delay/1
  raw_val/1 -> MATLAB Function/2(raw_val)
  Unit Delay/1 -> Cast To Double1/1
  freq_cut/1 -> Cast To Double/1
  Cast To Double/1 -> MATLAB Function/3(freq_cut)
  Cast To Double1/1 -> MATLAB Function/1(prev_val)

== system torch_zdof_sim/POS_HOLD CONTROLLER/Vertical speed controller/Vertical position controller ==
  cur_alt : Inport
  tar_z : Inport  Port=2
  P_alt : Inport  Port=3
  Altitude PID : slpidlib/PID Controller  Controller=P  Form=Ideal  TimeDomain=Discrete-time  UseExternalTs=off  SampleTime=framePeriod_s  IntegratorMethod=Forward Euler  FilterMethod=Forward Euler  ControllerParametersSource=external  P=0  I=0  UseKiTs=off  D=0  UseExternalDerivativeSource=off  N=100  UseFilter=off  TunerSelectOption=Frequency Response Based  ZeroCross=off  InitialConditionSource=internal  InitialConditionForIntegrator=0  InitialConditionForFilter=0  DifferentiatorICPrevScaledInput=0  ExternalReset=either  TrackingMode=off  Kt=1  LimitOutput=on  SatLimitsSource=internal  UpperSaturationLimit=Aircraft.Control.v_z_max  LowerSaturationLimit=-Aircraft.Control.v_z_max  LinearizeAsGain=on  AntiWindupMode=clamping  Kb=1  LimitIntegrator=off  UpperIntegratorSaturationLimit=inf  LowerIntegratorSaturationLimit=-inf  POutMin=[]  POutMax=[]  IOutMin=[]  IOutMax=[]  DOutMin=[]  DOutMax=[]  NOutMin=[]  NOutMax=[]  SumOutMin=[]  SumOutMax=[]  SaturationOutMin=[]  SaturationOutMax=[]  PParamMin=[]  PParamMax=[]  IParamMin=[]  IParamMax=[]  DParamMin=[]  DParamMax=[]  NParamMin=[]  NParamMax=[]  KbParamMin=[]  KbParamMax=[]  KtParamMin=[]  KtParamMax=[]  KbOutMin=[]  KbOutMax=[]  KtOutMin=[]  KtOutMax=[]  IntegratorOutMin=[]  IntegratorOutMax=[]  FilterOutMin=[]  FilterOutMax=[]  SumI1OutMin=[]  SumI1OutMax=[]  SumI2OutMin=[]  SumI2OutMax=[]  SumI3OutMin=[]  SumI3OutMax=[]  SumI4OutMin=[]  SumI4OutMax=[]  SumDOutMin=[]  SumDOutMax=[]  DifferentiatorOutMin=[]  DifferentiatorOutMax=[]  FilterDiffOutCoefMin=[]  FilterDiffOutCoefMax=[]  ReciprocalOutMin=[]  ReciprocalOutMax=[]  SumDenOutMin=[]  SumDenOutMax=[]  SumNumOutMin=[]  SumNumOutMax=[]  DivideOutMin=[]  DivideOutMax=[]  UdiffTsProdOutMin=[]  UdiffTsProdOutMax=[]  NTsProdOutMin=[]  NTsProdOutMax=[]  UintegralTsProdOutMin=[]  UintegralTsProdOutMax=[]  UngainTsProdOutMin=[]  UngainTsProdOutMax=[]  ClampingZeroOutDataTypeStr=Inherit: Inherit via back propagation  ClampingZeroOutMin=[]  ClampingZeroOutMax=[]  FilterDenConstantOutDataTypeStr=Inherit: Inherit via back propagation  FilterDenConstantOutMin=[]  FilterDenConstantOutMax=[]  PCopyOutDataTypeStr=Inherit: Inherit via back propagation  PCopyOutMin=[]  PCopyOutMax=[]  NCopyOutDataTypeStr=Inherit: Inherit via back propagation  NCopyOutMin=[]  NCopyOutMax=[]  IntegratorContinuousStateAttributes=''  IntegratorStateMustResolveToSignalObject=off  IntegratorRTWStateStorageClass=Auto  FilterContinuousStateAttributes=''  FilterStateMustResolveToSignalObject=off  FilterRTWStateStorageClass=Auto  ParallelPVariant=ExternalParameters  IdealPVariant=Disabled  IVariant=Disabled  DVariant=Disabled  IntegratorVariant=Disabled  SatVariant=Enabled  AWVariant=Disabled  PCopyVariant=Disabled  TRVariant=Disabled  FdbkBlocksVariant=Forward  IdealPFdbkVariant=Disabled  SatFdbkVariant=Disabled  DerivativeFilterVariant=Disabled  NVariant=Disabled  NCopyVariant=Disabled_SignalSpec  FilterICVariant=Disabled  IntegratorICVariant=Disabled  ExternalResetVariant=Disabled  TRSumVariant=Passthrough  SumFdbkVariant=Disabled  SumVariant=Passthrough_P  TsampFilterVariant=InternalTs  TsampNgainVariant=Passthrough  TsampIntegralVariant=Disabled_SignalSpec  ExternalSaturationOutDataTypeStr=Inherit: Same as second input  DerivativeSourceVariant=Disabled  PreIntVariant=InternalPreInt
  Sum3 : Sum  Inputs=|+-
  ve_z_cmd_mps : Outport
  wires:
  Altitude PID/1 -> ve_z_cmd_mps/1
  tar_z/1 -> Sum3/1  "target_z"
  cur_alt/1 -> Sum3/2
  Sum3/1 -> Altitude PID/1
  P_alt/1 -> Altitude PID/2

== system torch_zdof_sim/POS_HOLD CONTROLLER/Vertical speed controller/roll_D_DLPF ==
  raw_val : Inport
  freq_cut : Inport  Port=2
  Cast To Single : DataTypeConversion  OutDataTypeStr=single  SaturateOnIntegerOverflow=off  RndMeth=Floor
  Constant : Constant  Value=frameRate_hz  OutDataTypeStr=single
  MATLAB Function : MATLAB Function  TreatAsAtomicUnit=on
  Unit Delay : UnitDelay  SampleTime=-1  HasFrameUpgradeWarning=on
  filtered_val : Outport
  wires:
  freq_cut/1 -> MATLAB Function/3(freq_cut)
  MATLAB Function/1(filtered_val) -> Unit Delay/1, filtered_val/1
  Unit Delay/1 -> Cast To Single/1
  raw_val/1 -> MATLAB Function/2(raw_val)
  Constant/1 -> MATLAB Function/4(samp_freq)
  Cast To Single/1 -> MATLAB Function/1(prev_val)

== system torch_zdof_sim/POS_HOLD CONTROLLER/Vertical speed controller/set_tar_z when ve_z_cmd == 0 ==
  In1 : Inport
  Enable : EnablePort
  tar_z : Outport
  wires:
  In1/1 -> tar_z/1

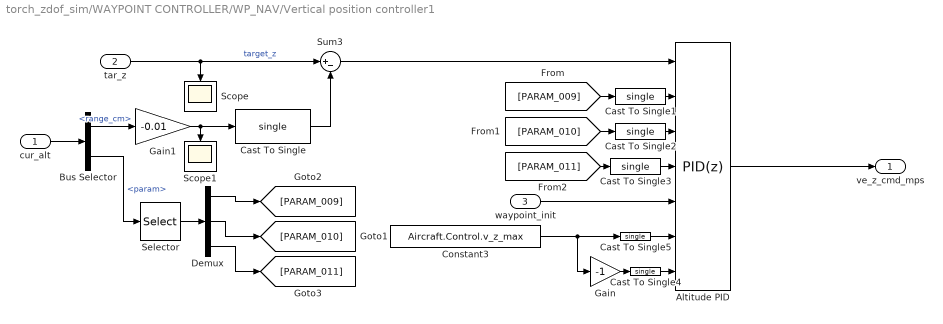
== system torch_zdof_sim/WAYPOINT CONTROLLER/WP_NAV/Vertical position controller1 ==
  cur_alt : Inport
  tar_z : Inport  Port=2
  waypoint_init : Inport  Port=3
  Altitude PID : slpidlib/PID Controller  Controller=PID  Form=Parallel  TimeDomain=Discrete-time  UseExternalTs=off  SampleTime=framePeriod_s  IntegratorMethod=Forward Euler  FilterMethod=Forward Euler  ControllerParametersSource=external  P=0  I=0  UseKiTs=off  D=0  UseExternalDerivativeSource=off  N=100  UseFilter=off  TunerSelectOption=Frequency Response Based  InitialConditionSource=internal  InitialConditionForIntegrator=0  InitialConditionForFilter=0  DifferentiatorICPrevScaledInput=0  ExternalReset=either  TrackingMode=off  Kt=1  LimitOutput=on  SatLimitsSource=external  UpperSaturationLimit=Aircraft.Control.v_z_max  LowerSaturationLimit=-Aircraft.Control.v_z_max  LinearizeAsGain=on  AntiWindupMode=clamping  Kb=1  LimitIntegrator=off  UpperIntegratorSaturationLimit=inf  LowerIntegratorSaturationLimit=-inf  POutMin=[]  POutMax=[]  IOutMin=[]  IOutMax=[]  DOutMin=[]  DOutMax=[]  NOutMin=[]  NOutMax=[]  SumOutMin=[]  SumOutMax=[]  SaturationOutMin=[]  SaturationOutMax=[]  PParamMin=[]  PParamMax=[]  IParamMin=[]  IParamMax=[]  DParamMin=[]  DParamMax=[]  NParamMin=[]  NParamMax=[]  KbParamMin=[]  KbParamMax=[]  KtParamMin=[]  KtParamMax=[]  KbOutMin=[]  KbOutMax=[]  KtOutMin=[]  KtOutMax=[]  IntegratorOutMin=[]  IntegratorOutMax=[]  FilterOutMin=[]  FilterOutMax=[]  SumI1OutMin=[]  SumI1OutMax=[]  SumI2OutMin=[]  SumI2OutMax=[]  SumI3OutMin=[]  SumI3OutMax=[]  SumI4OutMin=[]  SumI4OutMax=[]  SumDOutMin=[]  SumDOutMax=[]  DifferentiatorOutMin=[]  DifferentiatorOutMax=[]  FilterDiffOutCoefMin=[]  FilterDiffOutCoefMax=[]  ReciprocalOutMin=[]  ReciprocalOutMax=[]  SumDenOutMin=[]  SumDenOutMax=[]  SumNumOutMin=[]  SumNumOutMax=[]  DivideOutMin=[]  DivideOutMax=[]  UdiffTsProdOutMin=[]  UdiffTsProdOutMax=[]  NTsProdOutMin=[]  NTsProdOutMax=[]  UintegralTsProdOutMin=[]  UintegralTsProdOutMax=[]  UngainTsProdOutMin=[]  UngainTsProdOutMax=[]  ClampingZeroOutDataTypeStr=Inherit: Inherit via back propagation  ClampingZeroOutMin=[]  ClampingZeroOutMax=[]  FilterDenConstantOutDataTypeStr=Inherit: Inherit via back propagation  FilterDenConstantOutMin=[]  FilterDenConstantOutMax=[]  PCopyOutDataTypeStr=Inherit: Inherit via back propagation  PCopyOutMin=[]  PCopyOutMax=[]  NCopyOutDataTypeStr=Inherit: Inherit via back propagation  NCopyOutMin=[]  NCopyOutMax=[]  IntegratorContinuousStateAttributes=''  IntegratorStateMustResolveToSignalObject=off  IntegratorRTWStateStorageClass=Auto  FilterContinuousStateAttributes=''  FilterStateMustResolveToSignalObject=off  FilterRTWStateStorageClass=Auto  ParallelPVariant=ExternalParameters  IdealPVariant=Disabled  IVariant=ExternalParameters  DVariant=ExternalParameters  IntegratorVariant=Discrete  SatVariant=External  AWVariant=DiscClampingParallel  PCopyVariant=Disabled  TRVariant=Disabled  FdbkBlocksVariant=Forward  IdealPFdbkVariant=Disabled  SatFdbkVariant=Disabled  DerivativeFilterVariant=Differentiator  NVariant=Passthrough  NCopyVariant=Disabled_SignalSpec  FilterICVariant=InternalICsDifferentiator  IntegratorICVariant=InternalICs  ExternalResetVariant=ExternalReset  TRSumVariant=Passthrough  SumFdbkVariant=Disabled  SumVariant=Sum_PID  TsampFilterVariant=InternalTs  TsampNgainVariant=Passthrough  TsampIntegralVariant=Disabled_SignalSpec  ExternalSaturationOutDataTypeStr=Inherit: Same as second input  DerivativeSourceVariant=ErrorSignal  PreIntVariant=InternalPreInt
  Bus Selector : BusSelector  OutputSignals=Sensor Data.tfmini.range_cm,Telemetry Data.param
  Cast To Single{,1..5} (6 alike) : DataTypeConversion  OutDataTypeStr=single  SaturateOnIntegerOverflow=off  RndMeth=Floor
  Constant3 : Constant  Value=Aircraft.Control.v_z_max  OutDataTypeStr=double
  Demux : Demux  Outputs=3
  Gain : Gain  Gain=-1
  Gain1 : Gain  Gain=-0.01
  Scope : Scope
      settings: ActiveDisplayYMinimum=-1  ActiveDisplayYMaximum=1
  Scope1 : Scope
      settings: ActiveDisplayYMinimum=-1  ActiveDisplayYMaximum=1  DataLoggingVariableName=ScopeData4
  Selector : Selector  IndexMode=Zero-based  InputPortWidth=24  IndexOptions=Index vector (dialog)  Indices=[9 10 11]  OutputSizes=1
  Sum3 : Sum  Inputs=|+-
  ve_z_cmd_mps : Outport
  wires:
  Altitude PID/1 -> ve_z_cmd_mps/1
  tar_z/1 -> Scope/1, Sum3/1  "target_z"
  Constant3/1 -> Cast To Single5/1, Gain/1
  Bus Selector/2 -> Selector/1  "<param>"
  Selector/1 -> Demux/1
  cur_alt/1 -> Bus Selector/1
  Sum3/1 -> Altitude PID/1
  Demux/2 -> [PARAM_010]
  Demux/1 -> [PARAM_009]
  waypoint_init/1 -> Altitude PID/5
  Demux/3 -> [PARAM_011]
  [PARAM_009] -> Cast To Single1/1
  Cast To Single1/1 -> Altitude PID/2
  Cast To Single3/1 -> Altitude PID/4
  [PARAM_011] -> Cast To Single3/1
  [PARAM_010] -> Cast To Single2/1
  Cast To Single2/1 -> Altitude PID/3
  Gain/1 -> Cast To Single4/1
  Cast To Single4/1 -> Altitude PID/7
  Cast To Single5/1 -> Altitude PID/6
  Gain1/1 -> Scope1/1, Cast To Single/1
  Bus Selector/1 -> Gain1/1  "<range_cm>"
  Cast To Single/1 -> Sum3/2

== matlab function torch_zdof_sim/OUTER_TO_INNER_CONV/calc_body_throttle ==
  data: raw_thrust_vector input size=[3,1]; throttle output; hover_thr input; max_g_thrust input; gain input
function throttle = calc_body_throttle(raw_thrust_vector, hover_thr, max_g_thrust,gain)
    mag = norm(raw_thrust_vector);
    throttle = hover_thr + gain * (1 - hover_thr)*(mag - 1)/(max_g_thrust - 1);
    throttle = single(throttle);
end

== matlab function torch_zdof_sim/POS_HOLD CONTROLLER/Vertical speed controller/Pitch_D_DLPF/MATLAB Function ==
  data: prev_val input; raw_val input; filtered_val output; freq_cut input
function filtered_val = IIR_filt( prev_val,raw_val, freq_cut)
    fc = freq_cut/100;
    b = 2 - cos(2 * pi * fc) - sqrt((2 - cos(2 * pi * fc))^2 - 1);
    a = 1 - b;
    filtered_val = a * raw_val + b * prev_val;

== matlab function torch_zdof_sim/OUTER_TO_INNER_CONV/thrust_limit ==
  data: thrust_vector_raw input size=[3,1]; limited_vector output size=[3,1]; max_thrust input
function limited_vector = limit_thrust(thrust_vector_raw, max_thrust)
    % Limit the acceleration command to the max thrust achievable by the
    % aircraft. Should prioritize vertical thrust
    % Input:
    %           thrust_vector_raw - raw acceleration command
    %           max_thrust - max thrust by aircraft. In term of G
    limited_vector = single(thrust_vector_raw);
    mag = single(norm(thrust_vector_raw));
    % Ignore if the acc_cmd is already achieble
    if mag < max_thrust
        limited_vector = single(thrust_vector_raw);
    else
        if thrust_vector_raw(3) < -max_thrust
            limited_vector(3) = -max_thrust;
        end
        hor_acc = sqrt(max_thrust^2 - limited_vector(3)^2);
        limited_vector(1) = thrust_vector_raw(1) * hor_acc/mag;
        limited_vector(2) = thrust_vector_raw(2) * hor_acc/mag;
    end
    limited_vector = single(limited_vector);
end

== matlab function torch_zdof_sim/6DOF Low Fidelity/Friction ==
  data: weight input; F_command input; Vb input; output output; thresh input; x input
function output = fcn(weight, F_command, Vb, thresh, x)

Fz = weight + F_command;

%position limits
if abs(x(3))<=0.01 && Fz(3)>0
    output = [0;0;0];
    return;
elseif abs(x(3))>=1.2 && Fz(3)<0
    output = [0;0;0];
    return;
end

%friction
Cf = 2;
kinetic_friction = [0;0;Cf*Vb(3)];
if (abs(Fz(3)) < thresh) && (abs(Vb(3)) < 0.01)
    output = [0;0;0];
else
    output = Fz + (kinetic_friction.*-1);
end

== matlab function torch_zdof_sim/OUTER_TO_INNER_CONV/MATLAB Function ==
  data: base_weight input; hover_thr output; cable_kg_per_m input; C_t input; height input
function hover_thr = calc_hover_thrust(base_weight, cable_kg_per_m, C_t, height)
    hover_thr = (base_weight + cable_kg_per_m * height) * 9.81 / C_t;
    hover_thr = single(hover_thr);
end

== matlab function torch_zdof_sim/Stab_input_conversion/remap from min_spin to max1/remap1 ==
  data: raw_in input; norm_out output; in_min input; in_max input; out_min input; out_max input
function norm_out = remap(raw_in,in_min,in_max,out_min,out_max)
norm_out = (raw_in - in_min) * (out_max - out_min)/(in_max-in_min) + out_min;

== matlab function torch_zdof_sim/POS_HOLD_input_conversion/height_limiter ==
  data: vel_param_cmd input; vel_z_cmd output; h input
function vel_z_cmd = height_limiter(vel_param_cmd, h)

    if (vel_param_cmd == 0 && h <= 10)
        vel_z_cmd = -0.1;
    elseif (vel_param_cmd >= 0 && h <= 10)
        vel_z_cmd = 0;
    elseif (vel_param_cmd <= 0 && h >= 100)
        vel_z_cmd = 0;
    else
        vel_z_cmd = vel_param_cmd;
    end
    
end

== matlab function torch_zdof_sim/POS_HOLD CONTROLLER/Vertical speed controller/roll_D_DLPF/MATLAB Function ==
  data: prev_val input; raw_val input; filtered_val output; freq_cut input; samp_freq input
function filtered_val = IIR_filt( prev_val,raw_val, freq_cut, samp_freq)
    fc = freq_cut/samp_freq;
    b = 2 - cos(2 * pi * fc) - sqrt((2 - cos(2 * pi * fc))^2 - 1);
    a = 1 - b;
    filtered_val = a * raw_val + b * prev_val;

== matlab function torch_zdof_sim/WAYPOINT CONTROLLER/determine target/determine_current_tar_pos ==
  data: cur_target_pos output; fp_z input; wp_frame input
function cur_target_pos = determine_current_tar_pos(fp_z, wp_frame)
% WP reference frames
% 1 - relative to armed position
% 2 - who knows
% 3 - abosulute. Using lat, lon, alt
% 4 - cage frame. WP are relative to cage origin
    % if wp_frame == 3
    %     cur_target_pos = mission_item_to_ned(fp_x, fp_y, fp_z, home_lat_rad, home_lon_rad, home_alt);   
    % elseif wp_frame == 4
    %     r2d = 180 / pi;
    %     cage_origin = [33.2154770, -87.5436600, 0];
    %     cage_home_pos_lla = [home_lat_rad * r2d, home_lon_rad * r2d, 0];
    %     cage_home_pos_ned = single(lla_to_ned(cage_home_pos_lla, cage_origin));
    %     cur_target_pos = single([fp_x; -fp_y; -fp_z]) - cage_home_pos_ned;
    if wp_frame == 1
        cur_target_pos = single([0; 0; fp_z]);
    else
        cur_target_pos = single([0; 0; 0]);
    end
end

== matlab function torch_zdof_sim/WAYPOINT CONTROLLER/wp_completion_check/check_wp_reached ==
  data: target_pos input; reached output boolean; ned_pos input; Aircraft_Control_wp_radius input
function reached = check_wp_reached(target_pos, ned_pos, Aircraft_Control_wp_radius)

diff = target_pos - ned_pos;
reached = norm(diff) <= Aircraft_Control_wp_radius;
